simulink model "PalmSat_mono"  (R2017b)
settings: Solver=VariableStepAuto  StartTime=0.0  StopTime=20  RelTol=1e-3
values from neighbouring files (symbols this model uses):
  B = ModeloSatelite.B    [PalmSatModelScript.m]
  Kt = Kw/0.00684    (= 25.0525729951)    [PalmSatModelScript.m]
  Kw = 60*2*pi/2200    (= 0.171359599287)    [PalmSatModelScript.m]
  La = 74.4*10^-6    (= 7.44e-05)    [PalmSatModelScript.m]
  Ra = 0.225    [PalmSatModelScript.m]
undefined symbols (not defined in the file or in its folder): IA, IB, IC, J
settings Model: Creator=Gpiaia  LastModifiedBy=Gpiaia

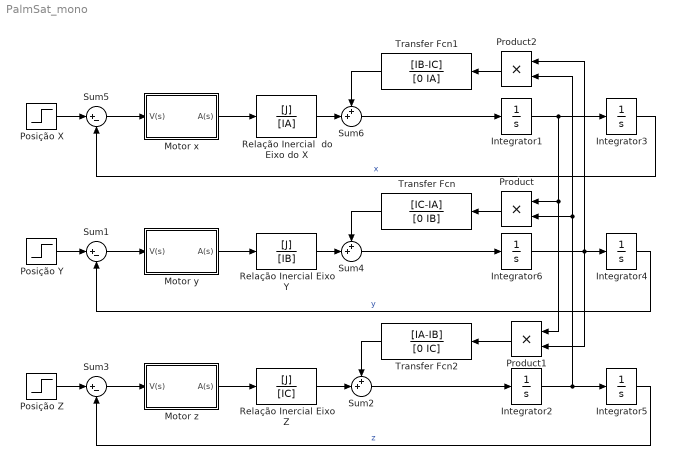
== system PalmSat_mono ==
  Integrator{1..6} (6 alike) : Integrator
  Motor x : Subsystem
  Motor y : Subsystem
  Motor z : Subsystem
  Posição X : Step  Time=5  After=0  SampleTime=0
  Posição Y : Step  Time=4  After=0  SampleTime=0
  Posição Z : Step  After=45  SampleTime=0
  Product : Product
  Product1 : Product
  Product2 : Product
  Relação Inercial Eixo Y : TransferFcn  Numerator=[J]  Denominator=[IB]
  Relação Inercial Eixo Z : TransferFcn  Numerator=[J]  Denominator=[IC]
  Relação Inercial  do Eixo do X : TransferFcn  Numerator=[J]  Denominator=[IA]
  Sum1 : Sum  Inputs=|+-
  Sum2 : Sum  Inputs=++|
  Sum3 : Sum  Inputs=|+-
  Sum4 : Sum  Inputs=++|
  Sum5 : Sum  Inputs=|+-
  Sum6 : Sum  Inputs=++|
  Transfer Fcn : TransferFcn  Numerator=[IC-IA]  Denominator=[0 IB]
  Transfer Fcn1 : TransferFcn  Numerator=[IB-IC]  Denominator=[0 IA]
  Transfer Fcn2 : TransferFcn  Numerator=[IA-IB]  Denominator=[0 IC]
  wires:
  Motor z/1(A(s)) -> Relação Inercial Eixo Z/1
  Transfer Fcn2/1 -> Sum2/1
  Transfer Fcn/1 -> Sum4/1
  Posição Z/1 -> Sum3/1
  Relação Inercial Eixo Y/1 -> Sum4/2
  Posição Y/1 -> Sum1/1
  Relação Inercial Eixo Z/1 -> Sum2/2
  Transfer Fcn1/1 -> Sum6/1
  Product2/1 -> Transfer Fcn1/1
  Product/1 -> Transfer Fcn/1
  Motor y/1(A(s)) -> Relação Inercial Eixo Y/1
  Integrator5/1 -> Sum3/2  "z"
  Integrator1/1 -> Integrator3/1, Product1/1, Product/1
  Posição X/1 -> Sum5/1
  Sum6/1 -> Integrator1/1
  Motor x/1(A(s)) -> Relação Inercial  do Eixo do X/1
  Sum1/1 -> Motor y/1(V(s))
  Sum3/1 -> Motor z/1(V(s))
  Sum2/1 -> Integrator2/1
  Product1/1 -> Transfer Fcn2/1
  Relação Inercial  do Eixo do X/1 -> Sum6/2
  Integrator3/1 -> Sum5/2  "x"
  Sum5/1 -> Motor x/1(V(s))
  Sum4/1 -> Integrator6/1
  Integrator4/1 -> Sum1/2  "y"
  Integrator2/1 -> Integrator5/1, Product2/2, Product/2
  Integrator6/1 -> Integrator4/1, Product1/2, Product2/1

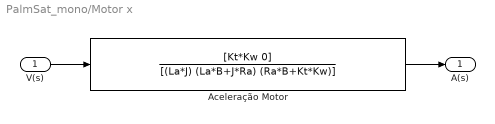
== system PalmSat_mono/Motor x ==
  V(s) : Inport
  Aceleração Motor : TransferFcn  Numerator=[Kt*Kw 0]  Denominator=[(La*J) (La*B+J*Ra) (Ra*B+Kt*Kw)]
  A(s) : Outport
  wires:
  V(s)/1 -> Aceleração Motor/1
  Aceleração Motor/1 -> A(s)/1

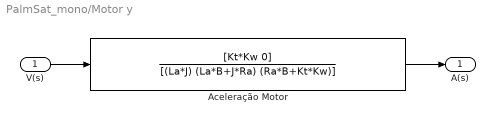
== system PalmSat_mono/Motor y ==
  V(s) : Inport
  Aceleração Motor : TransferFcn  Numerator=[Kt*Kw 0]  Denominator=[(La*J) (La*B+J*Ra) (Ra*B+Kt*Kw)]
  A(s) : Outport
  wires:
  V(s)/1 -> Aceleração Motor/1
  Aceleração Motor/1 -> A(s)/1

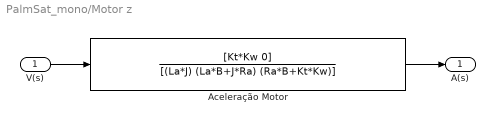
== system PalmSat_mono/Motor z ==
  V(s) : Inport
  Aceleração Motor : TransferFcn  Numerator=[Kt*Kw 0]  Denominator=[(La*J) (La*B+J*Ra) (Ra*B+Kt*Kw)]
  A(s) : Outport
  wires:
  V(s)/1 -> Aceleração Motor/1
  Aceleração Motor/1 -> A(s)/1
